simulink model "for_each_subsystem"  (R2014a)
settings: Solver=FixedStepDiscrete  StartTime=0.0  StopTime=10.0  FixedStep=0.1  RelTol=1e-3
settings Model: BufferReuse=off  Creator=yoshi12  LastModifiedBy=ts1413
settings OptimizationCC: BlockReduction=off  OptimizeBlockIOStorage=off  BufferReuse=off  GlobalBufferReuse=off  ExpressionFolding=off  LocalBlockOutputs=off  OptimizeModelRefInitCode=on  LifeSpan=1
settings RTWCC: SystemTargetFile=ert.tlc  GenCodeOnly=on  TemplateMakefile=ert_default_tmf  Description=Embedded Coder  ProcessScript=ert_make_rtw_hook
settings CodeAppCC: IgnoreCustomStorageClasses=off
settings ERTTargetCC: ParMdlRefBuildCompliant=on  CompOptLevelCompliant=on  ConcurrentExecutionCompliant=on  ERTFirstTimeCompliant=on  ModelStepFunctionPrototypeControlCompliant=on  CPPClassGenCompliant=on  InlinedParameterPlacement=Hierarchical  ERTCustomFileTemplate=example_file_process.tlc

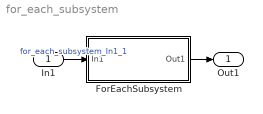
== system for_each_subsystem ==
  In1 : Inport
  ForEachSubsystem : Subsystem  TreatAsAtomicUnit=on
  Out1 : Outport
  wires:
  In1/1 -> ForEachSubsystem/1(In1)  "for_each_subsystem_In1_1"
  ForEachSubsystem/1(Out1) -> Out1/1

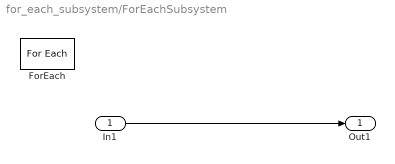
== system for_each_subsystem/ForEachSubsystem ==
  In1 : Inport  Partition=on  PartitionDimension=1  PartitionWidth=1
  ForEach : ForEach  DisableCoverage=on  IndexMode=One-based
  Out1 : Outport  ConcatenationDimension=1
  wires:
  In1/1 -> Out1/1
